simulink model "ADHW4p4"  (R2022a)
settings: Solver=VariableStepAuto  StartTime=0.0  StopTime=1800.0  RelTol=1e-3
settings Model: Creator=izacu  LastModifiedBy=izacu

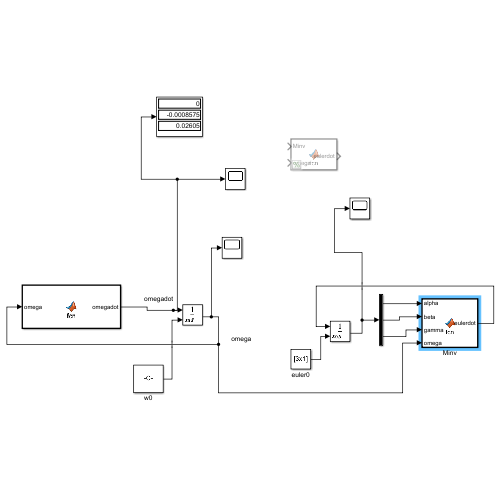
[thumbnail: Simulink's stored preview of the top-level diagram]
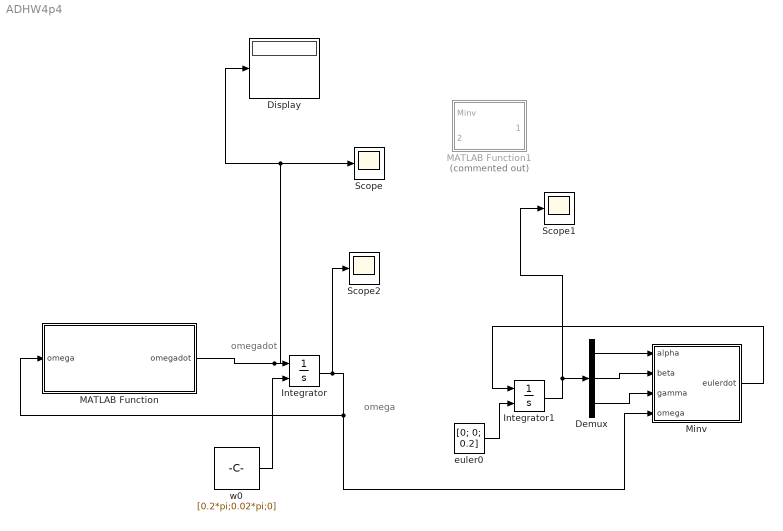
== system ADHW4p4 ==
  note: omegadot
  note: omega
  Demux : Demux  Outputs=3
  Display : Display
  Integrator : Integrator  InitialConditionSource=external
  Integrator1 : Integrator  InitialConditionSource=external
  MATLAB Function : MATLAB Function  TreatAsAtomicUnit=on
  MATLAB Function1 : MATLAB Function  Commented=on  TreatAsAtomicUnit=on
  Minv : MATLAB Function  TreatAsAtomicUnit=on
  Scope : Scope
  Scope1 : Scope
  Scope2 : Scope
  euler0 : Constant  Value=[0; 0; 0.2]
  w0 : Constant  Value=[0.2*pi;0.02*pi;0]
  wires:
  w0/1 -> Integrator/2
  MATLAB Function/1(omegadot) -> Scope/1, Display/1, Integrator/1
  Integrator/1 -> Scope2/1, Minv/4(omega), MATLAB Function/1(omega)
  euler0/1 -> Integrator1/2
  Integrator1/1 -> Scope1/1, Demux/1
  Demux/1 -> Minv/1(alpha)
  Demux/2 -> Minv/2(beta)
  Demux/3 -> Minv/3(gamma)
  Minv/1(eulerdot) -> Integrator1/1

== matlab function ADHW4p4/MATLAB Function ==
  data: omega input; omegadot output
function omegadot = fcn(omega)
J = [100 0 0;
    0 60 0;
    0 0 60];
omegadot = -inv(J)*[cross(omega,J*omega)];

== matlab function ADHW4p4/Minv ==
  data: alpha input; eulerdot output; beta input; gamma input; omega input
function eulerdot = fcn(alpha,beta,gamma,omega)

% Minv = (1/cos(beta))*[sin(gamma) cos(gamma) 0;
%     cos(beta)*cos(gamma) cos(beta)*sin(gamma) 0;
%     -sin(beta)*sin(gamma) -sin(beta)*cos(gamma) cos(beta)];

M = [cos(beta)*sin(gamma) cos(gamma) 0;
    cos(beta)*cos(gamma) -sin(gamma) 0;
    -sin(beta) 0 1];

eulerdot = M\omega;

== matlab function ADHW4p4/MATLAB Function1 ==
  data: Minv input; eulerdot output; omega input
function eulerdot = fcn(Minv,omega)

eulerdot = Minv*omega;
